simulink model "equations_dynamiques_synchrone"  (R2018b)
settings: Solver=VariableStepAuto  StartTime=0.0  StopTime=100  RelTol=1e-3
values from neighbouring files (symbols this model uses):
  alpha = 1    [Poteau_main.m]
  ca = 0.18    [Poteau_main.m]
  g = 9.81    [Poteau_main.m]
  Jt = M*Rw*Rw    (= 10.0188)    [Poteau_main.m]
  Lambdam = 0.0744    [Poteau_main.m]
  Ls = 0.0021    [Poteau_main.m]
  M = 92    [Poteau_main.m]
  Np = 52    [Poteau_main.m]
  Rs = 0.124    [Poteau_main.m]
  Rw = 0.33    [Poteau_main.m]
  s = tan(inc)    [Poteau_main.m]
libraries: simulink x2
settings Model: Creator=passeral  LastModifiedBy=poteaum

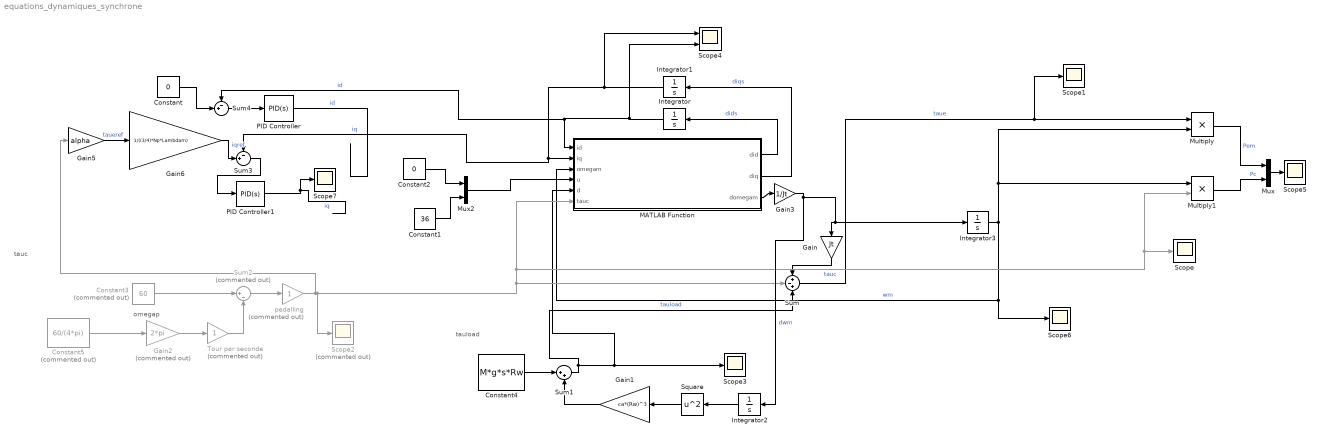
== system equations_dynamiques_synchrone ==
  note: tauload
  note: tauc
  note: omegap
  Constant : Constant  Value=0
  Constant1 : Constant  Value=36
  Constant2 : Constant  Value=0
  Constant3 : Constant  Commented=on  Value=60
  Constant4 : Constant  Value=M*g*s*Rw
  Constant5 : Constant  Commented=on  Value=60/(4*pi)
  Gain : Gain  Gain=Jt
  Gain1 : Gain  Gain=ca*(Rw)^3
  Gain2 : Gain  Commented=on  Gain=2*pi
  Gain3 : Gain  Gain=1/Jt
  Gain5 : Gain  Gain=alpha
  Gain6 : Gain  Gain=1/((3/4)*Np*Lambdam)
  Integrator : Integrator
  Integrator1 : Integrator
  Integrator2 : Integrator
  Integrator3 : Integrator  InitialCondition=1
  MATLAB Function : MATLAB Function  TreatAsAtomicUnit=on
  Multiply : Product
  Multiply1 : Product
  Mux : Mux  Inputs=2
  Mux2 : Mux  Inputs=2
  PID Controller : simulink/Continuous/PID Controller  Controller=PID  Form=Parallel  TimeDomain=Continuous-time  SampleTime=-1  IntegratorMethod=Forward Euler  FilterMethod=Forward Euler  ControllerParametersSource=internal  P=Rs  I=Rs^2/Ls  D=0  UseFilter=on  N=100  TunerSelectOption=Transfer Function Based (PID Tuner App)  InitialConditionSource=internal  InitialConditionForIntegrator=0  InitialConditionForFilter=0  DifferentiatorICPrevScaledInput=0  ExternalReset=none  TrackingMode=off  Kt=1  LimitOutput=off  UpperSaturationLimit=inf  LowerSaturationLimit=-inf  LinearizeAsGain=on  AntiWindupMode=none  Kb=1  POutMin=[]  POutMax=[]  IOutMin=[]  IOutMax=[]  DOutMin=[]  DOutMax=[]  NOutMin=[]  NOutMax=[]  SumOutMin=[]  SumOutMax=[]  SaturationOutMin=[]  SaturationOutMax=[]  PParamMin=[]  PParamMax=[]  IParamMin=[]  IParamMax=[]  DParamMin=[]  DParamMax=[]  NParamMin=[]  NParamMax=[]  KbParamMin=[]  KbParamMax=[]  KtParamMin=[]  KtParamMax=[]  KbOutMin=[]  KbOutMax=[]  KtOutMin=[]  KtOutMax=[]  IntegratorOutMin=[]  IntegratorOutMax=[]  FilterOutMin=[]  FilterOutMax=[]  SumI1OutMin=[]  SumI1OutMax=[]  SumI2OutMin=[]  SumI2OutMax=[]  SumI3OutMin=[]  SumI3OutMax=[]  SumI4OutMin=[]  SumI4OutMax=[]  SumDOutMin=[]  SumDOutMax=[]  DifferentiatorOutMin=[]  DifferentiatorOutMax=[]  FilterDiffOutCoefMin=[]  FilterDiffOutCoefMax=[]  ReciprocalOutMin=[]  ReciprocalOutMax=[]  SumDenOutMin=[]  SumDenOutMax=[]  SumNumOutMin=[]  SumNumOutMax=[]  DivideOutMin=[]  DivideOutMax=[]  IntegratorContinuousStateAttributes=''  IntegratorStateMustResolveToSignalObject=off  IntegratorRTWStateStorageClass=Auto  FilterContinuousStateAttributes=''  FilterStateMustResolveToSignalObject=off  FilterRTWStateStorageClass=Auto  ParallelPVariant=InternalParameters  IdealPVariant=Disabled  IVariant=InternalParameters  DVariant=InternalParameters  IntegratorVariant=Continuous  SatVariant=Disabled  AWVariant=Passthrough  PCopyVariant=Disabled  TRVariant=Disabled  FdbkBlocksVariant=Forward  IdealPFdbkVariant=Disabled  SatFdbkVariant=Disabled  DerivativeFilterVariant=ContFilter  NVariant=InternalParameters  NCopyVariant=Disabled  FilterICVariant=InternalICsFilter  IntegratorICVariant=InternalICs  ExternalResetVariant=Disabled  TRSumVariant=Passthrough  SumFdbkVariant=Disabled  SumVariant=Sum_PID
  PID Controller1 : simulink/Continuous/PID Controller  Controller=PID  Form=Parallel  TimeDomain=Continuous-time  SampleTime=-1  IntegratorMethod=Forward Euler  FilterMethod=Forward Euler  ControllerParametersSource=internal  P=Rs  I=Rs^2/Ls  D=0  UseFilter=on  N=100  TunerSelectOption=Transfer Function Based (PID Tuner App)  InitialConditionSource=internal  InitialConditionForIntegrator=0  InitialConditionForFilter=0  DifferentiatorICPrevScaledInput=0  ExternalReset=none  TrackingMode=off  Kt=1  LimitOutput=off  UpperSaturationLimit=inf  LowerSaturationLimit=-inf  LinearizeAsGain=on  AntiWindupMode=none  Kb=1  POutMin=[]  POutMax=[]  IOutMin=[]  IOutMax=[]  DOutMin=[]  DOutMax=[]  NOutMin=[]  NOutMax=[]  SumOutMin=[]  SumOutMax=[]  SaturationOutMin=[]  SaturationOutMax=[]  PParamMin=[]  PParamMax=[]  IParamMin=[]  IParamMax=[]  DParamMin=[]  DParamMax=[]  NParamMin=[]  NParamMax=[]  KbParamMin=[]  KbParamMax=[]  KtParamMin=[]  KtParamMax=[]  KbOutMin=[]  KbOutMax=[]  KtOutMin=[]  KtOutMax=[]  IntegratorOutMin=[]  IntegratorOutMax=[]  FilterOutMin=[]  FilterOutMax=[]  SumI1OutMin=[]  SumI1OutMax=[]  SumI2OutMin=[]  SumI2OutMax=[]  SumI3OutMin=[]  SumI3OutMax=[]  SumI4OutMin=[]  SumI4OutMax=[]  SumDOutMin=[]  SumDOutMax=[]  DifferentiatorOutMin=[]  DifferentiatorOutMax=[]  FilterDiffOutCoefMin=[]  FilterDiffOutCoefMax=[]  ReciprocalOutMin=[]  ReciprocalOutMax=[]  SumDenOutMin=[]  SumDenOutMax=[]  SumNumOutMin=[]  SumNumOutMax=[]  DivideOutMin=[]  DivideOutMax=[]  IntegratorContinuousStateAttributes=''  IntegratorStateMustResolveToSignalObject=off  IntegratorRTWStateStorageClass=Auto  FilterContinuousStateAttributes=''  FilterStateMustResolveToSignalObject=off  FilterRTWStateStorageClass=Auto  ParallelPVariant=InternalParameters  IdealPVariant=Disabled  IVariant=InternalParameters  DVariant=InternalParameters  IntegratorVariant=Continuous  SatVariant=Disabled  AWVariant=Passthrough  PCopyVariant=Disabled  TRVariant=Disabled  FdbkBlocksVariant=Forward  IdealPFdbkVariant=Disabled  SatFdbkVariant=Disabled  DerivativeFilterVariant=ContFilter  NVariant=InternalParameters  NCopyVariant=Disabled  FilterICVariant=InternalICsFilter  IntegratorICVariant=InternalICs  ExternalResetVariant=Disabled  TRSumVariant=Passthrough  SumFdbkVariant=Disabled  SumVariant=Sum_PID
  Scope{,1,3,5..7} (6 alike) : Scope
  Scope2 : Scope  Commented=on
  Scope4 : Scope  NumInputPorts=2
  Square : Math  Operator=square  OutputSignalType=real  SaturateOnIntegerOverflow=on
  Sum : Sum  Inputs=+-+
  Sum1 : Sum  Inputs=|++
  Sum2 : Sum  Commented=on  Inputs=|+-
  Sum3 : Sum  Inputs=-+|
  Sum4 : Sum  Inputs=-+|
  Tour par seconde : Gain  Commented=on
  "pedalling " : Gain  Commented=on
  wires:
  MATLAB Function/1(did) -> Integrator/1  "dids"
  MATLAB Function/2(diq) -> Integrator1/1  "diqs"
  MATLAB Function/3(domegam) -> Gain3/1
  Integrator3/1 -> MATLAB Function/3(omegam), Scope6/1, Multiply/2, Multiply1/1  "wm"
  Gain/1 -> Sum/1
  Sum/1 -> Scope1/1, Multiply/1  "taue"
  Integrator1/1 -> Scope4/1, MATLAB Function/2(iq), Sum3/1  "iq"
  Integrator2/1 -> Square/1
  Square/1 -> Gain1/1
  Gain1/1 -> Sum1/2
  Constant4/1 -> Sum1/1
  Sum1/1 -> Sum/3, MATLAB Function/5(d), Scope3/1  "tauload"
  Gain2/1 -> Tour par seconde/1
  Constant5/1 -> Gain2/1
  Constant3/1 -> Sum2/1
  Tour par seconde/1 -> Sum2/2
  Sum2/1 -> "pedalling "/1
  "pedalling "/1 -> Gain5/1, Scope2/1, Scope/1, Multiply1/2, MATLAB Function/6(tauc), Sum/2  "tauc"
  Gain3/1 -> Integrator2/1, Gain/1, Integrator3/1  "dwm"
  Multiply/1 -> Mux/1  "Pem"
  Multiply1/1 -> Mux/2  "Pc"
  Mux/1 -> Scope5/1
  PID Controller1/1 -> Scope7/1  "iq"
  Sum3/1 -> PID Controller1/1
  Gain6/1 -> Sum3/2  "iqref"
  Gain5/1 -> Gain6/1  "taueref"
  Constant/1 -> Sum4/2
  Sum4/1 -> PID Controller/1
  Integrator/1 -> Sum4/1, MATLAB Function/1(id), Scope4/2  "id"
  PID Controller/1 -> ?  "id"
  Mux2/1 -> MATLAB Function/4(u)
  Constant2/1 -> Mux2/1
  Constant1/1 -> Mux2/2

== matlab function equations_dynamiques_synchrone/MATLAB Function ==
  data: id input size=1; iq input size=1; omegam input size=1; u input size=2; did output size=1; d input size=1; diq output size=1; domegam output size=1; tauc input size=1
function [did, diq, domegam]  = Dynamiquesynchrone(id, iq, omegam,u, d, tauc)
% global Rs Ls Lambdam Np Jm 
Rs=0.124;   %R STATOR
Ls=0.0021;   %L Stator
Lambdam=0.0744; %Flux magnétique
Np=52;  %Nb poles
Jm=0.0028;  %Moment d'inertie moteur

% id=x(1);
% iq=x(2);
% omegam=x(3);
Vd = u(1); Vq = u(2);
tauload=d;
% xd = zeros(3,1);
did =Vd/Ls-(Rs/Ls)*id+(Np/2)*iq;
diq = Vq/Ls-(Rs/Ls)*iq-(Np/2)*id -(Np/2)*Lambdam;
domegam =((3*Np/4)*Lambdam*iq-tauload + tauc);
